simulink library "INT_PthLead_TrqCalc"  (R2016b)
settings: Solver=VariableStepAuto  StartTime=0.0  StopTime=10.0  RelTol=1e-3
settings Model: Creator=xuxingpei  LastModifiedBy=xuxingpei

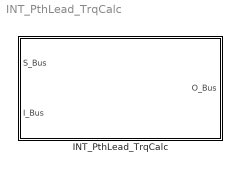
== system INT_PthLead_TrqCalc ==
  INT_PthLead_TrqCalc : Subsystem

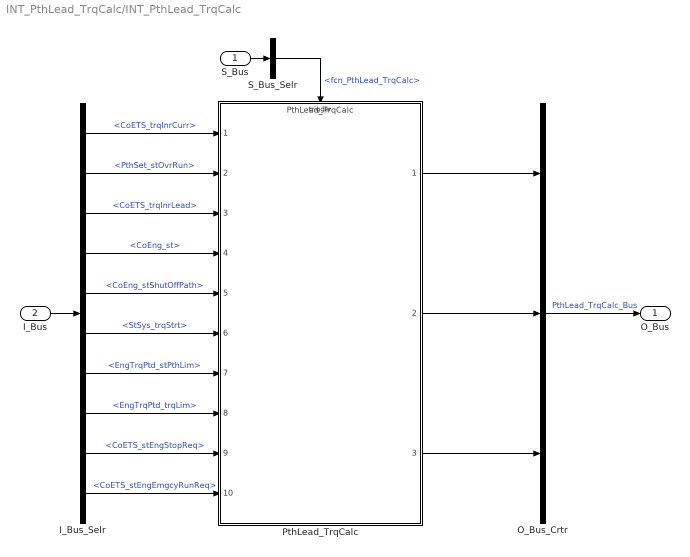
== system INT_PthLead_TrqCalc/INT_PthLead_TrqCalc ==
  S_Bus : Inport
  I_Bus : Inport  Port=2
  I_Bus_Selr : BusSelector  OutputSignals=CoETS_trqInrCurr,PthSet_stOvrRun,CoETS_trqInrLead,CoEng_st,CoEng_stShutOffPath,StSys_trqStrt,EngTrqPtd_stPthLim,EngTrqPtd_trqLim,CoETS_stEngStopReq,CoETS_stEngEmgcyRunReq
  O_Bus_Crtr : BusCreator  Inputs=3
  PthLead_TrqCalc : ModelReference  ModelNameDialog=PthLead_TrqCalc  SimulationMode=Normal  ModelReferenceVersion=1.8  TriggerPortName=function  TriggerPortTriggerType=function-call  TriggerPortStatesWhenEnabling=held
  S_Bus_Selr : BusSelector  OutputSignals=fcn_PthLead_TrqCalc
  O_Bus : Outport
  wires:
  S_Bus_Selr/1 -> PthLead_TrqCalc/Trigger  "<fcn_PthLead_TrqCalc>"
  S_Bus/1 -> S_Bus_Selr/1
  I_Bus/1 -> I_Bus_Selr/1
  I_Bus_Selr/1 -> PthLead_TrqCalc/1  "<CoETS_trqInrCurr>"
  I_Bus_Selr/2 -> PthLead_TrqCalc/2  "<PthSet_stOvrRun>"
  I_Bus_Selr/3 -> PthLead_TrqCalc/3  "<CoETS_trqInrLead>"
  I_Bus_Selr/4 -> PthLead_TrqCalc/4  "<CoEng_st>"
  I_Bus_Selr/5 -> PthLead_TrqCalc/5  "<CoEng_stShutOffPath>"
  I_Bus_Selr/6 -> PthLead_TrqCalc/6  "<StSys_trqStrt>"
  I_Bus_Selr/7 -> PthLead_TrqCalc/7  "<EngTrqPtd_stPthLim>"
  I_Bus_Selr/8 -> PthLead_TrqCalc/8  "<EngTrqPtd_trqLim>"
  I_Bus_Selr/9 -> PthLead_TrqCalc/9  "<CoETS_stEngStopReq>"
  I_Bus_Selr/10 -> PthLead_TrqCalc/10  "<CoETS_stEngEmgcyRunReq>"
  O_Bus_Crtr/1 -> O_Bus/1  "PthLead_TrqCalc_Bus"
  PthLead_TrqCalc/1 -> O_Bus_Crtr/1
  PthLead_TrqCalc/2 -> O_Bus_Crtr/2
  PthLead_TrqCalc/3 -> O_Bus_Crtr/3
